simulink library "bcm"  (R2021b)
settings: Solver=VariableStepAuto  StartTime=0.0  StopTime=10.0  RelTol=1e-3
undefined symbols (not defined in the file or in its folder): ENUM_ANTITHEFT_ALARM, ENUM_ANTITHEFT_ARM, ENUM_ANTITHEFT_DISARM, ENUM_ANTITHEFT_WAIT, ENUM_GEARPOSNTOCAN_P, ENUM_PDKEYRAWLULOCK_INUNLOCK, ENUM_PDKEYRAWPS_INPS, ENUM_POWERSTA_ON, ENUM_POWERSTA_READY, ENUM_POWERSTA_STANDBY, FALSE, KBCM_ALMBrightnessDark_enum, KBCM_AmbBlue_enum, KBCM_AmbBreathT_ms, KBCM_AmbGreen_enum, KBCM_AmbRed_enum, KBCM_Antitheft_enum_ovrdflg, KBCM_Antitheft_enum_ovrdval, KBCM_APMDoorCtrlSta_flg_ovrdflg, KBCM_APMDoorCtrlSta_flg_ovrdval, KBCM_DelayTSW_flg, KBCM_DiagFLTC_mA, KBCM_DiagFMHT_s, KBCM_DiagFRTC_mA, KBCM_DiagRLTC_mA, KBCM_DiagRRTC_mA, KBCM_DrAPMRetryTimes_cnt, KBCM_DrOpenWdwOT_s, KBCM_DrOpenWdwReady_s, KBCM_ESSOffT_ms, KBCM_ESSOnT_ms, KBCM_IVIRstHoldT_ms, KBCM_IVIRstTriggerT_ms, KBCM_ONDelayT_ms, KBCM_ReDetectT_K, KBCM_RmLampKeep_min, KBCM_RmLpKeyInT_s, KBCM_RmLpKeyMissT_s, KBCM_SlpDebounceTime_s, KBCM_SPTGDetectT_sec, KBCM_SPTGLeave_flg, KBCM_SPTGLeftBound_cm, KBCM_SPTGLeftBoundOut_cm, KBCM_SPTGLowerBound_cm, KBCM_SPTGLowerBoundOut_cm, KBCM_SPTGRightBound_cm, KBCM_SPTGRightBoundOut_cm, KBCM_SPTGTOut_K, KBCM_SPTGUpperBound_cm, KBCM_SPTGUpperBoundOut_cm, KBCM_SPTGWaitDKC_sec, KBCM_TrunSWKeepTime3_s, KBCM_TrunSWKeepTime5_s, KBCM_TrunSWKeepTime7_s, KBCM_USSDis_cm, KBCM_USSFilterT_K, KBCM_WaitAPMPwr_K, KBCM_WdwManualDetT_s, MIN2SEC, TRUE ... (+1)
libraries: simulink x151, hcu_lib x5
(part 3 of 8)

== system bcm/BCM/BCM/APM_Door ==
  task_time_s : Inport
  VINP_OpenDrOpenWdoSW_flg : Inport  Port=2
  VINP_LDrvControlCommand_pct : Inport  Port=3
  VINP_LDrvValWdwOpened_pct : Inport  Port=4
  VINP_DrDoorSW_flg : Inport  Port=5
  VINP_LPasControlCommand_pct : Inport  Port=6
  VINP_LPasValWdwOpened_pct : Inport  Port=7
  VINP_PsDoorSW_flg : Inport  Port=8
  VINP_LRLDControlCommand_pct : Inport  Port=9
  VINP_LRLDValWdwOpened_pct : Inport  Port=10
  VINP_RLDoorSW_flg : Inport  Port=11
  VINP_LRRDControlCommand_pct : Inport  Port=12
  VINP_LRRDValWdwOpened_pct : Inport  Port=13
  VINP_RRDoorSW_flg : Inport  Port=14
  VINP_FlashAPMDoorControlSta_flg : Inport  Port=15
  BCMInitial : Inport  Port=16
  VINP_CANMsgValidIVI2_flg : Inport  Port=17
  VINP_CANMsgValidGWZoneDR1_flg : Inport  Port=18
  VINP_CANMsgValidGWZoneFR1_flg : Inport  Port=19
  Constant{,5..6,15} (4 alike) : Constant  Value=KBCM_WdwManualDetT_s
  Constant{1,3,7,10} (4 alike) : Constant  Value=KBCM_DrOpenWdwReady_s
  Constant{2,8,11,14} (4 alike) : Constant  Value=KBCM_WaitAPMPwr_K
  Constant{4,9,12..13} (4 alike) : Constant  Value=KBCM_DrOpenWdwOT_s
  Constant16 : Constant  Value=KBCM_APMDoorCtrlSta_flg_ovrdflg
  Constant17 : Constant  Value=KBCM_APMDoorCtrlSta_flg_ovrdval
  Constant{18..21} (4 alike) : Constant  Value=KBCM_DrAPMRetryTimes_cnt
  Data Type Conversion : DataTypeConversion  OutDataTypeStr=single
  Detect Increase : simulink/Logic and Bit Operations/Detect Increase  vinit=0.0  OutDataTypeStr=boolean
  DoorAPM : Subsystem
  DoorAPM1 : Subsystem
  DoorAPM2 : Subsystem
  DoorAPM3 : Subsystem
  NOT : Logic  Operator=NOT  AllPortsSameDT=off  OutDataTypeStr=boolean
  Switch : Switch  Criteria=u2 ~= 0
  Switch1 : Switch  Criteria=u2 ~= 0
  Switch9 : Switch  Criteria=u2 > Threshold
  Terminator{,1..3} (4 alike) : Terminator
  Unit Delay2 : UnitDelay  InitialCondition=1  SampleTime=-1  HasFrameUpgradeWarning=on
  VBCM_LDrvCtrlCmd_pct : Outport
  VBCM_LPasCtrlCmd_pct : Outport  Port=2
  VBCM_LRLDCtrlCmd_pct : Outport  Port=3
  VBCM_LRRDCtrlCmd_pct : Outport  Port=4
  VBCM_APMDoorControlSta_flg : Outport  Port=5
  wires:
  NOT/1 -> Switch/1
  VINP_OpenDrOpenWdoSW_flg/1 -> Detect Increase/1
  Detect Increase/1 -> Switch/2
  VINP_FlashAPMDoorControlSta_flg/1 -> Switch9/3
  Unit Delay2/1 -> NOT/1, Switch/3
  Switch/1 -> Switch9/1
  Switch9/1 -> Switch1/3, Unit Delay2/1
  task_time_s/1 -> Data Type Conversion/1
  [task_time_s] -> DoorAPM/1(task_time_s)
  [task_time_s] -> DoorAPM1/1(task_time_s)
  [task_time_s] -> DoorAPM2/1(task_time_s)
  [task_time_s] -> DoorAPM3/1(task_time_s)
  DoorAPM/1(CtrlCmd_pct) -> VBCM_LDrvCtrlCmd_pct/1  "VBCM_LDrvCtrlCmd_pct"
  DoorAPM1/1(CtrlCmd_pct) -> VBCM_LPasCtrlCmd_pct/1  "VBCM_LPasCtrlCmd_pct"
  DoorAPM2/1(CtrlCmd_pct) -> VBCM_LRLDCtrlCmd_pct/1  "VBCM_LRLDCtrlCmd_pct"
  DoorAPM3/1(CtrlCmd_pct) -> VBCM_LRRDCtrlCmd_pct/1  "VBCM_LRRDCtrlCmd_pct"
  DoorAPM/2(CtrlCmdReady_flg) -> Terminator/1  "VBCM_LDrvCtrlCmdReady_flg"
  DoorAPM1/2(CtrlCmdReady_flg) -> Terminator1/1  "VBCM_LPasCtrlCmdReady_flg"
  DoorAPM2/2(CtrlCmdReady_flg) -> Terminator2/1  "VBCM_LRLDCtrlCmdReady_flg"
  DoorAPM3/2(CtrlCmdReady_flg) -> Terminator3/1  "VBCM_LRRDCtrlCmdReady_flg"
  Switch1/1 -> [VBCM_APMDoorControlSta_flg], VBCM_APMDoorControlSta_flg/1  "VBCM_APMDoorControlSta_flg"
  Constant16/1 -> Switch1/2
  Constant17/1 -> Switch1/1
  VINP_CANMsgValidIVI2_flg/1 -> [VINP_CANMsgValidIVI2_flg]
  VINP_CANMsgValidGWZoneDR1_flg/1 -> [VINP_CANMsgValidGWZoneDR1_flg]
  VINP_CANMsgValidGWZoneFR1_flg/1 -> [VINP_CANMsgValidGWZoneFR1_flg]
  [VINP_CANMsgValidGWZoneFR1_flg] -> DoorAPM/12(CANMsgValidGWZoneFR1)
  [VINP_CANMsgValidGWZoneDR1_flg] -> DoorAPM/11(CANMsgValidGWZoneDR1)
  [VBCM_APMDoorControlSta_flg] -> DoorAPM/5(APMDoorControlSta_flg)
  Constant8/1 -> DoorAPM/6(WaitAPMPwr_K)
  Constant9/1 -> DoorAPM/7(DrOpenWdwOT_s)
  Constant7/1 -> DoorAPM/8(DrOpenWdwReady_s)
  Constant18/1 -> DoorAPM/13(KBCM_DrAPMRetryTimes_cnt)
  Constant/1 -> DoorAPM/9(KBCM_WdwManualDetT_K)
  [VINP_CANMsgValidIVI2_flg] -> DoorAPM/10(CANMsgValidIVI2)
  VINP_DrDoorSW_flg/1 -> DoorAPM/2(DoorSW_flg)
  VINP_LDrvControlCommand_pct/1 -> DoorAPM/3(ControlCommand_pct)
  VINP_LDrvValWdwOpened_pct/1 -> DoorAPM/4(ValWdwOpened_pct)
  [VINP_CANMsgValidGWZoneDR1_flg] -> DoorAPM1/11(CANMsgValidGWZoneDR1)
  [VINP_CANMsgValidGWZoneFR1_flg] -> DoorAPM1/12(CANMsgValidGWZoneFR1)
  [VBCM_APMDoorControlSta_flg] -> DoorAPM1/5(APMDoorControlSta_flg)
  Constant11/1 -> DoorAPM1/6(WaitAPMPwr_K)
  Constant12/1 -> DoorAPM1/7(DrOpenWdwOT_s)
  Constant10/1 -> DoorAPM1/8(DrOpenWdwReady_s)
  Constant5/1 -> DoorAPM1/9(KBCM_WdwManualDetT_K)
  [VINP_CANMsgValidIVI2_flg] -> DoorAPM1/10(CANMsgValidIVI2)
  Constant19/1 -> DoorAPM1/13(KBCM_DrAPMRetryTimes_cnt)
  VINP_PsDoorSW_flg/1 -> DoorAPM1/2(DoorSW_flg)
  VINP_LPasControlCommand_pct/1 -> DoorAPM1/3(ControlCommand_pct)
  VINP_LPasValWdwOpened_pct/1 -> DoorAPM1/4(ValWdwOpened_pct)
  [VINP_CANMsgValidGWZoneDR1_flg] -> DoorAPM2/11(CANMsgValidGWZoneDR1)
  [VINP_CANMsgValidGWZoneFR1_flg] -> DoorAPM2/12(CANMsgValidGWZoneFR1)
  [VBCM_APMDoorControlSta_flg] -> DoorAPM2/5(APMDoorControlSta_flg)
  Constant2/1 -> DoorAPM2/6(WaitAPMPwr_K)
  Constant13/1 -> DoorAPM2/7(DrOpenWdwOT_s)
  Constant1/1 -> DoorAPM2/8(DrOpenWdwReady_s)
  Constant6/1 -> DoorAPM2/9(KBCM_WdwManualDetT_K)
  [VINP_CANMsgValidIVI2_flg] -> DoorAPM2/10(CANMsgValidIVI2)
  Constant20/1 -> DoorAPM2/13(KBCM_DrAPMRetryTimes_cnt)
  VINP_RLDoorSW_flg/1 -> DoorAPM2/2(DoorSW_flg)
  VINP_LRLDControlCommand_pct/1 -> DoorAPM2/3(ControlCommand_pct)
  VINP_LRLDValWdwOpened_pct/1 -> DoorAPM2/4(ValWdwOpened_pct)
  [VINP_CANMsgValidGWZoneDR1_flg] -> DoorAPM3/11(CANMsgValidGWZoneDR1)
  [VINP_CANMsgValidGWZoneFR1_flg] -> DoorAPM3/12(CANMsgValidGWZoneFR1)
  [VBCM_APMDoorControlSta_flg] -> DoorAPM3/5(APMDoorControlSta_flg)
  Constant14/1 -> DoorAPM3/6(WaitAPMPwr_K)
  Constant4/1 -> DoorAPM3/7(DrOpenWdwOT_s)
  Constant3/1 -> DoorAPM3/8(DrOpenWdwReady_s)
  Constant15/1 -> DoorAPM3/9(KBCM_WdwManualDetT_K)
  [VINP_CANMsgValidIVI2_flg] -> DoorAPM3/10(CANMsgValidIVI2)
  Constant21/1 -> DoorAPM3/13(KBCM_DrAPMRetryTimes_cnt)
  VINP_RRDoorSW_flg/1 -> DoorAPM3/2(DoorSW_flg)
  VINP_LRRDControlCommand_pct/1 -> DoorAPM3/3(ControlCommand_pct)
  VINP_LRRDValWdwOpened_pct/1 -> DoorAPM3/4(ValWdwOpened_pct)
  Data Type Conversion/1 -> [task_time_s]
  BCMInitial/1 -> Switch9/2

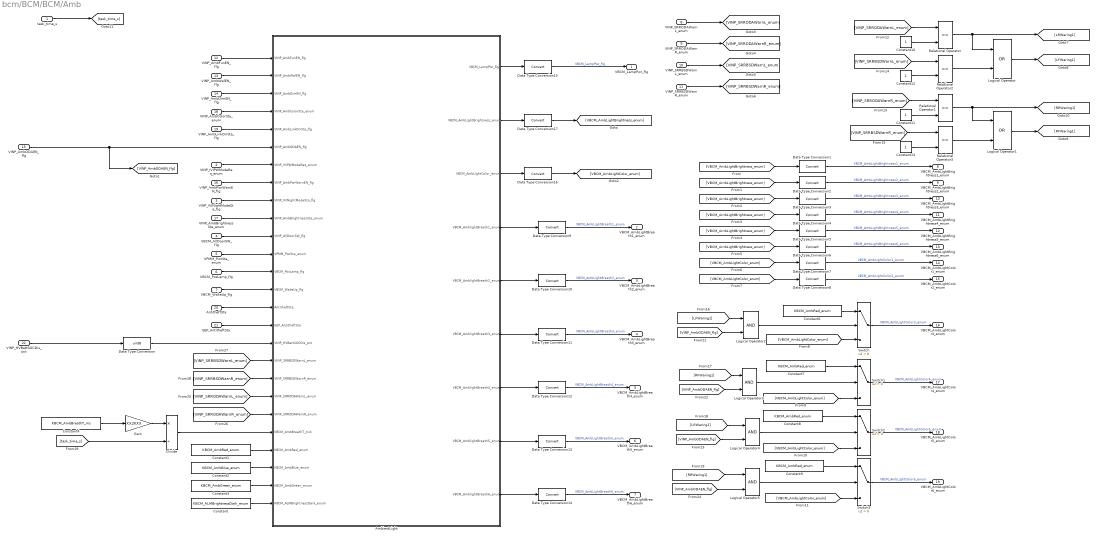
== system bcm/BCM/BCM/Amb ==
  task_time_s : Inport
  VINP_IVIPWModeReq_enum : Inport  Port=2
  VINP_IVINightModeSta_flg : Inport  Port=3
  VBCM_AllDoorSW_flg : Inport  Port=4
  VPMM_PwrSta_enum : Inport  Port=5
  VBCM_PosLamp_flg : Inport  Port=6
  VBCM_WakeUp_flg : Inport  Port=7
  VINP_SRRODAWarnL_enum : Inport  Port=8
  VINP_SRRODAWarnR_enum : Inport  Port=9
  VINP_SRRBSDWarnL_enum : Inport  Port=10
  VINP_SRRBSDWarnR_enum : Inport  Port=11
  VINP_AmbFunEN_flg : Inport  Port=12
  VINP_AmbWelEN_flg : Inport  Port=13
  VINP_AmbDimEN_flg : Inport  Port=14
  VINP_AmbODAEN_flg : Inport  Port=15
  VINP_AmbPwrWarnEN_flg : Inport  Port=16
  VINP_AmbBrightnessSta_enum : Inport  Port=17
  VINP_AmbColorSta_enum : Inport  Port=18
  VINP_AmbLinkDriSta_flg : Inport  Port=19
  AntitheftSta : Inport  Port=20
  EEP_AntitheftSta : Inport  Port=21
  VINP_HVBattSOCDis_pct : Inport  Port=22
  AmbientLight : Stateflow chart  TreatAsAtomicUnit=on
      settings: PortSchema="{\"entries\":[{\"content\":{\"sides\":[{\"content\":{\"connectorIds\":[\"In4\",\"In1\",\"In3\",\"In2\",\"In11\",\"In6\",\"In12\",\"In8\",\"In15\",\"In10\",\"In17\",\"In18\",\"In16\",\"In19\",\"In20\",\"In21\",\"In22\",\"In23\",\"In24\",\"In25\",\"In26\",\"In14\",\"In9\",\"In13\",\"In7\",\"In5\"]},\"type\":\"ConnectorPlacement.EquallySpacedRectSide\",\"uuid\":\"e6ddbb92-6bab-4ee4-8600-41e59bb8ed99\"},{\"content\":{\"connectorIds\":[\"Out1\",\"Out2\",\"Out3\",\"Out4\",\"Out5\",\"Out6\",\"Out7\",\"Out8\",\"Out9\"],\"side\":\"RIGHT\"},\"type\":\"ConnectorPlacement.EquallySpacedRectSide\",\"uuid\":\"8a02ea17-d632-4a57-b5aa-65195147745e\"},{\"content\":{\"side\":\"TOP\"},\"type\":\"ConnectorPlacement.EquallySpacedRectSide\",\"uuid\":\"3394b4a4-a92c-4aad-9aa4-5f4e7dfad0c8\"}]},\"type\":\"ConnectorPlacement.EquallySpacedConnector\",\"uuid\":\"350d749b-651a-4475-8984-e64d423840e0\"}],\"packageUris\":[\"http://schema.mathworks.com/mf0/Connector/R2020b\"],\"version\":\"1.0\"}"
  Constant : Constant  Value=KBCM_ALMBrightnessDark_enum  OutDataTypeStr=uint8
  Constant{1,6..9} (5 alike) : Constant  Value=KBCM_AmbRed_enum  OutDataTypeStr=uint8
  Constant{10..13} (4 alike) : Constant
  Constant2 : Constant  Value=KBCM_AmbBlue_enum  OutDataTypeStr=uint8
  Constant3 : Constant  Value=KBCM_AmbGreen_enum  OutDataTypeStr=uint8
  Constant4 : Constant  Value=KBCM_AmbBreathT_ms
  Data Type Conversion : DataTypeConversion  OutDataTypeStr=uint8
  Data Type Conversion{1..17} (17 alike) : DataTypeConversion
  Divide : Product  Inputs=*/
  Gain : Gain  Gain=XX2KXX
  Logical Operator : Logic  Operator=OR  AllPortsSameDT=off  OutDataTypeStr=boolean
  Logical Operator1 : Logic  Operator=OR  AllPortsSameDT=off  OutDataTypeStr=boolean
  Logical Operator{2..5} (4 alike) : Logic  AllPortsSameDT=off  OutDataTypeStr=boolean
  Relational Operator{,1..3} (4 alike) : RelationalOperator  Operator===  OutDataTypeStr=boolean  RndMeth=Simplest
  Switch{,1..3} (4 alike) : Switch  Criteria=u2 > Threshold
  VBCM_LampPwr_flg : Outport
  VBCM_AmbLightBreath1_enum : Outport  Port=2
  VBCM_AmbLightBreath2_enum : Outport  Port=3
  VBCM_AmbLightBreath3_enum : Outport  Port=4
  VBCM_AmbLightBreath4_enum : Outport  Port=5
  VBCM_AmbLightBreath5_enum : Outport  Port=6
  VBCM_AmbLightBreath6_enum : Outport  Port=7
  VBCM_AmbLightBrightness1_enum : Outport  Port=8
  VBCM_AmbLightBrightness2_enum : Outport  Port=9
  VBCM_AmbLightBrightness3_enum : Outport  Port=10
  VBCM_AmbLightBrightness4_enum : Outport  Port=11
  VBCM_AmbLightBrightness5_enum : Outport  Port=12
  VBCM_AmbLightBrightness6_enum : Outport  Port=13
  VBCM_AmbLightColor1_enum : Outport  Port=14
  VBCM_AmbLightColor2_enum : Outport  Port=15
  VBCM_AmbLightColor3_enum : Outport  Port=16
  VBCM_AmbLightColor4_enum : Outport  Port=17
  VBCM_AmbLightColor5_enum : Outport  Port=18
  VBCM_AmbLightColor6_enum : Outport  Port=19
  wires:
  [RRWaring1] -> Logical Operator5/1
  VINP_SRRBSDWarnR_enum/1 -> [VINP_SRRBSDWarnR_enum]
  Relational Operator3/1 -> Logical Operator1/2
  [VBCM_AmbLightColor_enum] -> Switch/3
  Relational Operator/1 -> [LRWaring1], Logical Operator/1
  [VINP_AmbODAEN_flg] -> Logical Operator3/2
  [VINP_SRRBSDWarnR_enum] -> Relational Operator3/1
  Constant8/1 -> Switch2/1
  [VBCM_AmbLightBrightness_enum] -> Data Type Conversion2/1
  Constant11/1 -> Relational Operator1/2
  Constant10/1 -> Relational Operator/2
  [VBCM_AmbLightBrightness_enum] -> Data Type Conversion4/1
  [VINP_AmbODAEN_flg] -> Logical Operator4/2
  Logical Operator4/1 -> Switch2/2
  [VINP_SRRBSDWarnL_enum] -> Relational Operator2/1
  AmbientLight/3(VBCM_AmbLightColor_enum) -> Data Type Conversion16/1
  [VINP_SRRODAWarnL_enum] -> AmbientLight/25(VINP_SRRODAWarnL_enum)
  [RFWaring1] -> Logical Operator3/1
  [VINP_SRRODAWarnR_enum] -> AmbientLight/26(VINP_SRRODAWarnR_enum)
  [VINP_AmbODAEN_flg] -> Logical Operator2/2
  Switch3/1 -> VBCM_AmbLightColor6_enum/1  "VBCM_AmbLightColor6_enum"
  VINP_SRRODAWarnR_enum/1 -> [VINP_SRRODAWarnR_enum]
  [LFWaring1] -> Logical Operator2/1
  [VBCM_AmbLightColor_enum] -> Switch1/3
  [VINP_SRRBSDWarnL_enum] -> AmbientLight/23(VINP_SRRBSDWarnL_enum)
  [VBCM_AmbLightBrightness_enum] -> Data Type Conversion6/1
  VBCM_PosLamp_flg/1 -> AmbientLight/16(VBCM_PosLamp_flg)
  VINP_SRRODAWarnL_enum/1 -> [VINP_SRRODAWarnL_enum]
  Constant1/1 -> AmbientLight/9(KBCM_AmbRed_enum)
  Logical Operator5/1 -> Switch3/2
  [VBCM_AmbLightColor_enum] -> Switch3/3
  Switch1/1 -> VBCM_AmbLightColor4_enum/1  "VBCM_AmbLightColor4_enum"
  Logical Operator3/1 -> Switch1/2
  Relational Operator1/1 -> Logical Operator1/1, [RRWaring1]
  VBCM_WakeUp_flg/1 -> AmbientLight/19(VBCM_WakeUp_flg)
  [VINP_SRRBSDWarnR_enum] -> AmbientLight/24(VINP_SRRBSDWarnR_enum)
  [VINP_SRRODAWarnR_enum] -> Relational Operator1/1
  Constant9/1 -> Switch3/1
  AmbientLight/8(VBCM_AmblightBreath5_enum) -> Data Type Conversion13/1
  AmbientLight/1(VBCM_LampPwr_flg) -> Data Type Conversion15/1
  Constant2/1 -> AmbientLight/13(KBCM_AmbBlue_enum)
  Constant13/1 -> Relational Operator3/2
  Constant3/1 -> AmbientLight/7(KBCM_AmbGreen_enum)
  Constant6/1 -> Switch/1
  AmbientLight/9(VBCM_AmblightBreath6_enum) -> Data Type Conversion14/1
  [VBCM_AmbLightColor_enum] -> Switch2/3
  [VBCM_AmbLightBrightness_enum] -> Data Type Conversion3/1
  VINP_SRRBSDWarnL_enum/1 -> [VINP_SRRBSDWarnL_enum]
  [VBCM_AmbLightBrightness_enum] -> Data Type Conversion5/1
  AmbientLight/7(VBCM_AmblightBreath4_enum) -> Data Type Conversion12/1
  Relational Operator2/1 -> Logical Operator/2
  AmbientLight/6(VBCM_AmblightBreath3_enum) -> Data Type Conversion11/1
  Logical Operator1/1 -> [RFWaring1]
  Logical Operator/1 -> [LFWaring1]
  Constant7/1 -> Switch1/1
  [VBCM_AmbLightColor_enum] -> Data Type Conversion7/1
  [VBCM_AmbLightColor_enum] -> Data Type Conversion8/1
  [VINP_SRRODAWarnL_enum] -> Relational Operator/1
  EEP_AntitheftSta/1 -> AmbientLight/21(EEP_AntitheftSta)
  Logical Operator2/1 -> Switch/2
  VINP_HVBattSOCDis_pct/1 -> Data Type Conversion/1
  Constant12/1 -> Relational Operator2/2
  Switch/1 -> VBCM_AmbLightColor3_enum/1  "VBCM_AmbLightColor3_enum"
  [VINP_AmbODAEN_flg] -> Logical Operator5/2
  Switch2/1 -> VBCM_AmbLightColor5_enum/1  "VBCM_AmbLightColor5_enum"
  AntitheftSta/1 -> AmbientLight/20(AntitheftSta)
  [LRWaring1] -> Logical Operator4/1
  VPMM_PwrSta_enum/1 -> AmbientLight/18(VPMM_PwrSta_enum)
  VBCM_AllDoorSW_flg/1 -> AmbientLight/17(VINP_AllDoorSW_flg)
  AmbientLight/5(VBCM_AmblightBreath2_enum) -> Data Type Conversion10/1
  [VBCM_AmbLightBrightness_enum] -> Data Type Conversion1/1
  AmbientLight/4(VBCM_AmblightBreath1_enum) -> Data Type Conversion9/1
  Constant/1 -> AmbientLight/5(KBCM_ALMBrightnessDark_enum)
  [task_time_s] -> Divide/2
  Gain/1 -> Divide/1
  Constant4/1 -> Gain/1
  Divide/1 -> AmbientLight/14(KBCM_AmbBreathT_tick)
  task_time_s/1 -> [task_time_s]
  VINP_AmbFunEN_flg/1 -> AmbientLight/4(VINP_AmbFunEN_flg)
  VINP_AmbWelEN_flg/1 -> AmbientLight/1(VINP_AmbWelEN_flg)
  VINP_AmbDimEN_flg/1 -> AmbientLight/3(VINP_AmbDimEN_flg)
  VINP_AmbColorSta_enum/1 -> AmbientLight/2(VINP_AmbColorSta_enum)
  VINP_AmbLinkDriSta_flg/1 -> AmbientLight/11(VINP_AmbLinkDriSta_flg)
  VINP_AmbODAEN_flg/1 -> [VINP_AmbODAEN_flg], AmbientLight/6(VINP_AmbODAEN_flg)
  VINP_IVIPWModeReq_enum/1 -> AmbientLight/12(VINP_IVIPWModeReq_enum)
  VINP_AmbPwrWarnEN_flg/1 -> AmbientLight/8(VINP_AmbPwrWarnEN_flg)
  VINP_IVINightModeSta_flg/1 -> AmbientLight/15(VINP_IVINightModeSta_flg)
  VINP_AmbBrightnessSta_enum/1 -> AmbientLight/10(VINP_AmbBrightnessSta_enum)
  Data Type Conversion/1 -> AmbientLight/22(VINP_HVBattSOCDis_pct)
  Data Type Conversion1/1 -> VBCM_AmbLightBrightness1_enum/1  "VBCM_AmbLightBrightness1_enum"
  Data Type Conversion2/1 -> VBCM_AmbLightBrightness2_enum/1  "VBCM_AmbLightBrightness2_enum"
  Data Type Conversion3/1 -> VBCM_AmbLightBrightness3_enum/1  "VBCM_AmbLightBrightness3_enum"
  Data Type Conversion4/1 -> VBCM_AmbLightBrightness4_enum/1  "VBCM_AmbLightBrightness4_enum"
  Data Type Conversion5/1 -> VBCM_AmbLightBrightness5_enum/1  "VBCM_AmbLightBrightness5_enum"
  Data Type Conversion6/1 -> VBCM_AmbLightBrightness6_enum/1  "VBCM_AmbLightBrightness6_enum"
  Data Type Conversion7/1 -> VBCM_AmbLightColor1_enum/1  "VBCM_AmbLightColor1_enum"
  Data Type Conversion8/1 -> VBCM_AmbLightColor2_enum/1  "VBCM_AmbLightColor2_enum"
  Data Type Conversion9/1 -> VBCM_AmbLightBreath1_enum/1  "VBCM_AmbLightBreath1_enum"
  Data Type Conversion10/1 -> VBCM_AmbLightBreath2_enum/1  "VBCM_AmbLightBreath2_enum"
  Data Type Conversion11/1 -> VBCM_AmbLightBreath3_enum/1  "VBCM_AmbLightBreath3_enum"
  Data Type Conversion12/1 -> VBCM_AmbLightBreath4_enum/1  "VBCM_AmbLightBreath4_enum"
  Data Type Conversion13/1 -> VBCM_AmbLightBreath5_enum/1  "VBCM_AmbLightBreath5_enum"
  Data Type Conversion14/1 -> VBCM_AmbLightBreath6_enum/1  "VBCM_AmbLightBreath6_enum"
  Data Type Conversion15/1 -> VBCM_LampPwr_flg/1  "VBCM_LampPwr_flg"
  Data Type Conversion16/1 -> [VBCM_AmbLightColor_enum]
  AmbientLight/2(VBCM_AmbLightBrightness_enum) -> Data Type Conversion17/1
  Data Type Conversion17/1 -> [VBCM_AmbLightBrightness_enum]

== system bcm/BCM/BCM/AntiTheft ==
  VINP_PCommandToBCM_enum : Inport
  VPMM_PwrSta_enum : Inport  Port=2
  VINP_HoodSW_flg : Inport  Port=3
  VINP_TailgateSW_flg : Inport  Port=4
  VINP_DrDoorSW_flg : Inport  Port=5
  VINP_PsDoorSW_flg : Inport  Port=6
  VINP_RLDoorSW_flg : Inport  Port=7
  VINP_RRDoorSW_flg : Inport  Port=8
  VINP_DrLockSta_flg : Inport  Port=9
  VINP_ReDoorLock_enum : Inport  Port=10
  VINP_VehSpeed_kph : Inport  Port=11
  VBCM_fVIGHandle_flg : Inport  Port=12
  VBCM_FlashAntitheft_enum : Inport  Port=13
  VINP_APSOpenPTG_flg : Inport  Port=14
  VINP_FlashCountAlarm_enum : Inport  Port=15
  VINP_CANMsgValidGWZoneDR1_flg : Inport  Port=16
  VINP_CANMsgValidGWZoneFR1_flg : Inport  Port=17
  VINP_CANMsgValidIVI1_flg : Inport  Port=18
  VINP_IVILockSoundSWSta_flg : Inport  Port=19
  Antitheft__override : Subsystem
  Chart : Stateflow chart  TreatAsAtomicUnit=on
  Data Type Conversion : DataTypeConversion  OutDataTypeStr=uint8
  Data Type Conversion1 : DataTypeConversion  OutDataTypeStr=boolean
  Logical Operator : Logic  Operator=OR  Inputs=4  AllPortsSameDT=off  OutDataTypeStr=boolean
  Switch : Switch  Criteria=u2 ~= 0
  Unit Delay : UnitDelay  SampleTime=-1  HasFrameUpgradeWarning=on
  VIG_Decoder : MATLAB Function  TreatAsAtomicUnit=on
  VBCM_ATCtrl_enum : Outport
  VBCM_ATActCtrl_enum : Outport  Port=2
  VBCM_ATAlarm_flg : Outport  Port=3
  VBCM_AntitheftSta_enum : Outport  Port=4
  VBCM_TailgateRemote_enum : Outport  Port=5
  VBCM_HornCtrl_flg : Outport  Port=6
  VBCM_AllDoorSW_flg : Outport  Port=7
  VBCM_BCMDoorLockSta_flg : Outport  Port=8
  VBCM_AntitehftSeatFlod_flg : Outport  Port=9
  VBCM_HoodSW_flg : Outport  Port=10
  VBCM_TailgateSW_flg : Outport  Port=11
  VBCM_DrDoorSW_flg : Outport  Port=12
  VBCM_PsDoorSW_flg : Outport  Port=13
  VBCM_RLDoorSW_flg : Outport  Port=14
  VBCM_RRDoorSW_flg : Outport  Port=15
  VBCM_CountAlarm_enum : Outport  Port=16
  VBCM_LockAlarm_enum : Outport  Port=17
  wires:
  VBCM_fVIGHandle_flg/1 -> Chart/13(fVIGHandle)  "VBCM_fVIGHandle_flg"
  VINP_RRDoorSW_flg/1 -> [RRDoorSW]
  VINP_ReDoorLock_enum/1 -> VIG_Decoder/1(VINP_ReDoorLock_enum)
  Chart/2(ATLockCtrl) -> VBCM_ATActCtrl_enum/1  "VBCM_ATActCtrl_enum"
  Chart/1(ATCtrl) -> VBCM_ATCtrl_enum/1  "VBCM_ATCtrl_enum"
  VINP_PCommandToBCM_enum/1 -> Chart/1(P_CommandtoBCM)
  VINP_RLDoorSW_flg/1 -> [RLDoorSW]
  Chart/3(ATAlarm) -> VBCM_ATAlarm_flg/1  "VBCM_ATAlarm_flg"
  VINP_PsDoorSW_flg/1 -> [PsDoorSW]
  VINP_VehSpeed_kph/1 -> Chart/12(VehSpeed)  "VINP_VehSpeed_kph"
  Logical Operator/1 -> [VBCM_AllDoorSW_flg]  "VBCM_AllDoorSW_flg"
  VINP_DrDoorSW_flg/1 -> [DrDoorSW]
  VINP_HoodSW_flg/1 -> [HoodSW]
  VIG_Decoder/1(VIG_Cmd) -> Data Type Conversion/1
  Data Type Conversion/1 -> Chart/11(VIG_Cmd)  "VBCM_VIGCommand_enum"
  [VBCM_AllDoorSW_flg] -> VBCM_AllDoorSW_flg/1  "VBCM_AllDoorSW_flg"
  Chart/4(AntitheftSta) -> Antitheft__override/1(In1)  "VBCM_AntitheftSta_enum"
  Chart/5(TailgateRemote) -> VBCM_TailgateRemote_enum/1  "VBCM_TailgateRemote_enum"
  Chart/6(HornCtrl) -> VBCM_HornCtrl_flg/1  "VBCM_HornCtrl_flg"
  Chart/7(AntitheftSeatFlod) -> VBCM_AntitehftSeatFlod_flg/1  "VBCM_AntitheftSeatFlod_flg"
  Antitheft__override/1(Out1) -> VBCM_AntitheftSta_enum/1  "VBCM_AntitheftSta_enum"
  VINP_APSOpenPTG_flg/1 -> Chart/15(APSOpenPTG)  "VINP_APSOpenPTG_flg"
  VINP_TailgateSW_flg/1 -> [TailgateSW]
  [DrDoorSW] -> Logical Operator/1
  [PsDoorSW] -> Logical Operator/2
  [RLDoorSW] -> Logical Operator/3
  [RRDoorSW] -> Logical Operator/4
  VINP_DrLockSta_flg/1 -> [DrLockSta]
  [DrLockSta] -> VBCM_BCMDoorLockSta_flg/1  "VBCM_BCMDoorLockSta_flg"
  [HoodSW] -> VBCM_HoodSW_flg/1  "VBCM_HoodSW_flg"
  [TailgateSW] -> VBCM_TailgateSW_flg/1  "VBCM_TailgateSW_flg"
  [DrDoorSW] -> VBCM_DrDoorSW_flg/1  "VBCM_DrDoorSW_flg"
  [PsDoorSW] -> VBCM_PsDoorSW_flg/1  "VBCM_PsDoorSW_flg"
  [RLDoorSW] -> VBCM_RLDoorSW_flg/1  "VBCM_RLDoorSW_flg"
  [RRDoorSW] -> VBCM_RRDoorSW_flg/1  "VBCM_RRDoorSW_flg"
  VPMM_PwrSta_enum/1 -> Chart/2(PwrSta)
  VBCM_FlashAntitheft_enum/1 -> Chart/14(VBCM_FlashAntitheft_enum)
  [DrDoorSW] -> Chart/6(DrDoorSW)
  [TailgateSW] -> Chart/5(TailgateSW)
  [PsDoorSW] -> Chart/7(PsDoorSW)
  [HoodSW] -> Chart/4(HoodSW)
  [RRDoorSW] -> Chart/9(RRDoorSW)
  [RLDoorSW] -> Chart/8(RLDoorSW)
  [DrLockSta] -> Chart/10(DrLockSta)
  [VBCM_AllDoorSW_flg] -> Chart/3(AllDoorSW)
  VINP_FlashCountAlarm_enum/1 -> Chart/16(VINP_FlashCountAlarm_enum)
  VINP_CANMsgValidGWZoneDR1_flg/1 -> Chart/17(VINP_CANMsgValidGWZoneDR1_flg)
  VINP_CANMsgValidGWZoneFR1_flg/1 -> Chart/18(VINP_CANMsgValidGWZoneFR1_flg)
  Chart/8(CountAlarm) -> VBCM_CountAlarm_enum/1  "VBCM_CountAlarm_enum"
  VINP_IVILockSoundSWSta_flg/1 -> Switch/1
  Switch/1 -> Data Type Conversion1/1, Unit Delay/1
  VINP_CANMsgValidIVI1_flg/1 -> Switch/2
  Unit Delay/1 -> Switch/3
  Chart/9(VBCM_LockAlarm_enum) -> VBCM_LockAlarm_enum/1  "VBCM_LockAlarm_enum"
  Data Type Conversion1/1 -> Chart/19(IVI_Lock_SoundSW_Sta)

== system bcm/BCM/BCM/BCM_WAKE_MODULE ==
  note: SIMULINK_BASED
  note: STATEFLOW_BASED
  note: The initial value of this uint dealy is "1"
  VBCM_HoodSW_flg : Inport
  VBCM_TailgateSW_flg : Inport  Port=2
  VBCM_CTDLockSW_flg : Inport  Port=3
  VBCM_TailgateHDSW_flg : Inport  Port=4
  VBCM_AntitheftSta_enum : Inport  Port=5
  VBCM_AllDoorSW_flg : Inport  Port=6
  VBCM_HornCtrl_flg : Inport  Port=7
  VBCM_DoorLockIND_flg : Inport  Port=8
  VINP_BrakeSWGPIO_flg : Inport  Port=9
  VBCM_PosLamp_flg : Inport  Port=10
  VBCM_LBSD_flg : Inport  Port=11
  VBCM_RBSD_flg : Inport  Port=12
  VBCM_LTurnLP_flg : Inport  Port=13
  VBCM_RTurnLP_flg : Inport  Port=14
  VBCM_MirrorCtrl_enum : Inport  Port=15
  VBCM_RoomLampH_flg : Inport  Port=16
  task_time_s : Inport  Port=17
  VINP_FlashHoodSW_flg : Inport  Port=18
  VINP_FlashTailgateSW_flg : Inport  Port=19
  VINP_FlashCTDLockSW_flg : Inport  Port=20
  VINP_FlashTailgateHDSW_flg : Inport  Port=21
  Chart : Stateflow chart  TreatAsAtomicUnit=on
  Compare To Constant : simulink/Logic and Bit Operations/Compare To Constant  relop=>  const=0  OutDataTypeStr=boolean
  Constant : Constant  Value=TRUE
  Constant1 : Constant  Commented=on  Value=TRUE
  Constant2 : Constant  Value=KBCM_SlpDebounceTime_s
  Constant5 : Constant  Commented=on  Value=KBCM_SlpDebounceTime_s
  Data Type Conversion : DataTypeConversion
  Detect Change : simulink/Logic and Bit Operations/Detect Change  vinit=0  OutDataTypeStr=boolean
  Detect Increase{,1..4} (5 alike) : simulink/Logic and Bit Operations/Detect Increase  vinit=0.0  OutDataTypeStr=boolean
  From : From  Commented=on  GotoTag=VBCM_SleepReq_flg
  From1 : From  Commented=on  GotoTag=VBCM_SlpConditionMeet_flg
  From2 : From  Commented=on  GotoTag=VBCM_SlpConditionMeet_flg
  From4 : From  Commented=on  GotoTag=task_time_s
  Goto : Goto  Commented=on  GotoTag=VBCM_SleepReq_flg
  Goto11 : Goto  Commented=on  GotoTag=VBCM_WakeUp_flg
  GreaterThan{,1..3} (4 alike) : RelationalOperator  Operator=>  OutDataTypeStr=boolean  RndMeth=Simplest
  GreaterThanOrEqual : RelationalOperator  Commented=on  OutDataTypeStr=boolean  RndMeth=Simplest
  Logical Operator : Logic  Operator=OR  Inputs=16  AllPortsSameDT=off  OutDataTypeStr=boolean
  Logical Operator{1,6..9} (5 alike) : Logic  AllPortsSameDT=off  OutDataTypeStr=boolean
  Logical Operator10 : Logic  Operator=NOT  AllPortsSameDT=off  OutDataTypeStr=boolean
  Logical Operator2 : Logic  Commented=on  AllPortsSameDT=off  OutDataTypeStr=boolean
  Logical Operator3 : Logic  Commented=on  Operator=NOT  AllPortsSameDT=off  OutDataTypeStr=boolean
  Logical Operator4 : Logic  Operator=NOT  AllPortsSameDT=off  OutDataTypeStr=boolean
  Logical Operator5 : Logic  Commented=on  Operator=NOT  AllPortsSameDT=off  OutDataTypeStr=boolean
  Switch : Switch  Commented=on  Criteria=u2 > Threshold
  Timer : hcu_lib/Basic_Blocks/Timer  Commented=on
  Udelay_Init_ONE : UnitDelay  Commented=on  InitialCondition=1  SampleTime=-1  HasFrameUpgradeWarning=on
  Unit Delay : UnitDelay  SampleTime=-1  HasFrameUpgradeWarning=on
  VBCM_SleepReq_flg : Outport
  VBCM_WakeUp_flg : Outport  Port=2
  wires:
  VBCM_DoorLockIND_flg/1 -> Logical Operator/8
  VBCM_LBSD_flg/1 -> Logical Operator/11
  VBCM_RoomLampH_flg/1 -> Logical Operator/16
  VBCM_RBSD_flg/1 -> Logical Operator/12
  VBCM_HornCtrl_flg/1 -> Logical Operator/7
  VBCM_AllDoorSW_flg/1 -> Detect Increase/1
  VBCM_RTurnLP_flg/1 -> Logical Operator/14
  Compare To Constant/1 -> Logical Operator/15
  VBCM_PosLamp_flg/1 -> Logical Operator/10
  VINP_BrakeSWGPIO_flg/1 -> Logical Operator/9
  VBCM_MirrorCtrl_enum/1 -> Compare To Constant/1
  VBCM_LTurnLP_flg/1 -> Logical Operator/13
  Detect Change/1 -> Logical Operator1/1
  VBCM_AntitheftSta_enum/1 -> Detect Change/1
  Constant5/1 -> GreaterThanOrEqual/2, Timer/4
  Timer/1 -> GreaterThanOrEqual/1
  Logical Operator/1 -> Logical Operator4/1
  Logical Operator1/1 -> Logical Operator/5
  Unit Delay/1 -> Logical Operator1/2
  Constant/1 -> Unit Delay/1
  Logical Operator4/1 -> [VBCM_SlpConditionMeet_flg]
  Switch/1 -> Logical Operator3/1, Goto/1  "VBCM_SleepReq_flg"
  Logical Operator2/1 -> Switch/2
  Constant1/1 -> Switch/1
  From/1 -> Udelay_Init_ONE/1
  GreaterThanOrEqual/1 -> Switch/3
  Udelay_Init_ONE/1 -> Logical Operator2/1
  Logical Operator5/1 -> Timer/2
  From2/1 -> Logical Operator2/2
  From1/1 -> Logical Operator5/1, Timer/1
  task_time_s/1 -> [task_time_s]
  From4/1 -> Timer/3
  VBCM_HoodSW_flg/1 -> [VBCM_HoodSW_flg]
  [VINP_FlashHoodSW_flg] -> GreaterThan/2
  GreaterThan/1 -> Logical Operator6/2
  Logical Operator6/1 -> Logical Operator/1
  [VBCM_HoodSW_flg] -> GreaterThan/1, Detect Increase4/1
  Detect Increase4/1 -> Logical Operator6/1
  VBCM_TailgateSW_flg/1 -> [VBCM_TailgateSW_flg]
  [VBCM_CTDLockSW_flg] -> Detect Increase2/1, GreaterThan2/1
  Detect Increase2/1 -> Logical Operator8/1
  GreaterThan2/1 -> Logical Operator8/2
  Logical Operator8/1 -> Logical Operator/3
  [VINP_FlashCTDLockSW_flg] -> GreaterThan2/2
  VBCM_CTDLockSW_flg/1 -> [VBCM_CTDLockSW_flg]
  [VBCM_TailgateHDSW_flg] -> Detect Increase3/1, GreaterThan3/1
  Detect Increase3/1 -> Logical Operator9/1
  [VINP_FlashTailgateHDSW_flg] -> GreaterThan3/2
  GreaterThan3/1 -> Logical Operator9/2
  VBCM_TailgateHDSW_flg/1 -> [VBCM_TailgateHDSW_flg]
  GreaterThan1/1 -> Logical Operator7/2
  Logical Operator7/1 -> Logical Operator/2
  [VINP_FlashTailgateSW_flg] -> GreaterThan1/2
  [VBCM_TailgateSW_flg] -> GreaterThan1/1, Detect Increase1/1
  Detect Increase1/1 -> Logical Operator7/1
  Logical Operator9/1 -> Logical Operator/4
  VINP_FlashHoodSW_flg/1 -> [VINP_FlashHoodSW_flg]
  VINP_FlashTailgateSW_flg/1 -> [VINP_FlashTailgateSW_flg]
  VINP_FlashCTDLockSW_flg/1 -> [VINP_FlashCTDLockSW_flg]
  VINP_FlashTailgateHDSW_flg/1 -> [VINP_FlashTailgateHDSW_flg]
  [task_time_s] -> Chart/2(task_time_s)
  Constant2/1 -> Chart/3(KBCM_SlpDebounceTime_s)
  [VBCM_SlpConditionMeet_flg] -> Chart/1(VBCM_SlpConditionMeet_flg)
  Logical Operator3/1 -> Goto11/1  "VBCM_WakeUp_flg"
  [VBCM_SleepReq_flg] -> VBCM_SleepReq_flg/1
  [VBCM_WakeUp_flg] -> VBCM_WakeUp_flg/1
  Logical Operator10/1 -> [VBCM_WakeUp_flg]
  Data Type Conversion/1 -> Logical Operator10/1, [VBCM_SleepReq_flg]  "VBCM_SleepReq_flg"
  Chart/1(VBCM_SleepReq_flg) -> Data Type Conversion/1
  Detect Increase/1 -> Logical Operator/6

== system bcm/BCM/BCM/CSW ==
  task_time_s : Inport
  VINP_CSWDimSwSta_flg : Inport  Port=2
  VINP_CSW2DimSwSta_flg : Inport  Port=3
  VINP_CSWPassSWSta_flg : Inport  Port=4
  VINP_CSW2PassSWSta_flg : Inport  Port=5
  VINP_CSWTurnSwSta_enum : Inport  Port=6
  VINP_CSW2TurnSwSta_enum : Inport  Port=7
  VINP_CSWFWipSwSta_enum : Inport  Port=8
  VINP_CSW2FWipSwSta_enum : Inport  Port=9
  VINP_CSWFWasSwSta_enum : Inport  Port=10
  VINP_CSW2FWasSwSta_enum : Inport  Port=11
  VINP_SASAngle_deg : Inport  Port=12
  VINP_TurnSwTimeSet_enum : Inport  Port=13
  VINP_LBeam_flg : Inport  Port=14
  VINP_CSW2RWIPWasSwSta_enum : Inport  Port=15
  VINP_CSWRWipIntSwSta_enum : Inport  Port=16
  VINP_CSWRWasSWSta_enum : Inport  Port=17
  Chart : Stateflow chart  TreatAsAtomicUnit=on
  Compare To Constant : simulink/Logic and Bit Operations/Compare To Constant  relop=<  const=3.0  OutDataTypeStr=boolean
  Compare To Constant1 : simulink/Logic and Bit Operations/Compare To Constant  relop=<  const=7  OutDataTypeStr=boolean
  Compare To Constant2 : simulink/Logic and Bit Operations/Compare To Constant  relop=<  const=3  OutDataTypeStr=boolean
  Compare To Constant3 : simulink/Logic and Bit Operations/Compare To Constant  relop=>=  const=5  OutDataTypeStr=boolean
  Compare To Constant4 : simulink/Logic and Bit Operations/Compare To Constant  relop=<  const=3.0  OutDataTypeStr=boolean
  Compare To Constant5 : simulink/Logic and Bit Operations/Compare To Constant  relop===  const=2  OutDataTypeStr=boolean
  Constant : Constant  Value=FALSE
  Constant1 : Constant  Value=45  OutDataTypeStr=int16
  Constant10 : Constant  Value=KBCM_TrunSWKeepTime5_s
  Constant11 : Constant  Value=2
  Constant12 : Constant  Value=KBCM_TrunSWKeepTime7_s
  Constant13 : Constant  Value=KBCM_TrunSWKeepTime3_s
  Constant2 : Constant  Value=TRUE
  Constant3 : Constant  Value=43  OutDataTypeStr=int16
  Constant4 : Constant  Value=FALSE
  Constant5 : Constant  Value=-45  OutDataTypeStr=int16
  Constant6 : Constant  Value=TRUE
  Constant7 : Constant  Value=-43  OutDataTypeStr=int16
  Constant8 : Constant  Value=FALSE
  Constant9 : Constant
  Data Type Conversion : DataTypeConversion  OutDataTypeStr=uint8
  Data Type Conversion1 : DataTypeConversion  OutDataTypeStr=uint16
  Data Type Conversion2 : DataTypeConversion  OutDataTypeStr=uint8
  Data Type Conversion3 : DataTypeConversion  OutDataTypeStr=uint8
  Detect Decrease : simulink/Logic and Bit Operations/Detect Decrease  vinit=0.0  OutDataTypeStr=boolean
  Detect Decrease1 : simulink/Logic and Bit Operations/Detect Decrease  vinit=0.0  OutDataTypeStr=boolean
  Detect Increase : simulink/Logic and Bit Operations/Detect Increase  vinit=0.0  OutDataTypeStr=boolean
  Detect Increase1 : simulink/Logic and Bit Operations/Detect Increase  vinit=0.0  OutDataTypeStr=boolean
  Divide : Product  Inputs=*/
  Logical Operator : Logic  Operator=NOT  AllPortsSameDT=off  OutDataTypeStr=boolean
  Logical Operator1 : Logic  AllPortsSameDT=off  OutDataTypeStr=boolean
  NOT : Logic  Operator=NOT  AllPortsSameDT=off  OutDataTypeStr=boolean
  OR : Logic  Operator=OR  AllPortsSameDT=off  OutDataTypeStr=boolean
  OR1 : Logic  Operator=OR  AllPortsSameDT=off  OutDataTypeStr=boolean
  Relational Operator : RelationalOperator  Operator=<  OutDataTypeStr=boolean  RndMeth=Simplest
  Relational Operator1 : RelationalOperator  Operator=>  OutDataTypeStr=boolean  RndMeth=Simplest
  Relational Operator2 : RelationalOperator  Operator=>  OutDataTypeStr=boolean  RndMeth=Simplest
  Relational Operator3 : RelationalOperator  Operator=<  OutDataTypeStr=boolean  RndMeth=Simplest
  Relational Operator4 : RelationalOperator  Operator===  OutDataTypeStr=boolean  RndMeth=Simplest
  Relational Operator5 : RelationalOperator  Operator===  OutDataTypeStr=boolean  RndMeth=Simplest
  Switch{,1..5} (6 alike) : Switch  Criteria=u2 > Threshold
  Switch{6..12} (7 alike) : Switch  Criteria=u2 ~= 0
  Unit Delay1 : UnitDelay  SampleTime=-1  HasFrameUpgradeWarning=on
  Unit Delay2 : UnitDelay  SampleTime=-1  HasFrameUpgradeWarning=on
  Unit Delay4 : UnitDelay  SampleTime=-1  HasFrameUpgradeWarning=on
  VBCM_DimSwSta_flg : Outport
  VBCM_PassSWSta_flg : Outport  Port=2
  VBCM_TurnSwSta_enum : Outport  Port=3
  VBCM_FWipSwSta_enum : Outport  Port=4
  VBCM_FWasSwSta_enum : Outport  Port=5
  VBCM_RWasSwSta_enum : Outport  Port=6
  VBCM_RWipIntSwSta_enum : Outport  Port=7
  wires:
  VINP_CSWDimSwSta_flg/1 -> OR/1
  Switch5/1 -> Switch4/3
  VINP_SASAngle_deg/1 -> Relational Operator1/2, Relational Operator2/2, Relational Operator3/2, Relational Operator/2
  Unit Delay2/1 -> Switch5/3
  Constant5/1 -> Relational Operator2/1
  Constant7/1 -> Relational Operator3/1
  Constant3/1 -> Relational Operator1/1
  Constant6/1 -> Switch4/1
  Relational Operator3/1 -> Switch5/2
  Detect Increase1/1 -> NOT/1
  Switch2/1 -> Unit Delay1/1, Detect Decrease/1
  Relational Operator1/1 -> Switch3/2
  Switch1/1 -> Switch/1
  VINP_CSW2TurnSwSta_enum/1 -> Compare To Constant3/1, Chart/1(VINP_CSW2TurnSwSta_enum)
  Switch6/1 -> [VBCM_WaitTimeSet_s]
  [LeftRelflg] -> Chart/2(LeftRelflg)
  Constant/1 -> Switch/3
  Constant1/1 -> Relational Operator/1
  Constant13/1 -> Switch7/3
  Switch7/1 -> Switch6/3
  Constant12/1 -> Switch7/1
  Constant10/1 -> Switch6/1
  [VINP_CSW2PassSWSta_flg] -> Detect Increase1/1
  Relational Operator2/1 -> Switch4/2
  OR/1 -> VBCM_DimSwSta_flg/1
  Constant8/1 -> Switch5/1
  Relational Operator/1 -> Switch2/2
  [RightRelflg] -> Chart/3(RightRelflg)
  Relational Operator5/1 -> Switch7/2
  Constant4/1 -> Switch3/1
  Detect Increase/1 -> Switch1/2
  Unit Delay1/1 -> Switch3/3
  Relational Operator4/1 -> Switch6/2
  Constant2/1 -> Switch2/1
  Switch4/1 -> Detect Decrease1/1, Unit Delay2/1
  VINP_CSW2FWipSwSta_enum/1 -> Compare To Constant1/1, Switch8/1
  VINP_CSW2DimSwSta_flg/1 -> Detect Increase/1
  VINP_TurnSwTimeSet_enum/1 -> [VINP_TurnSwTimeSet_enum]
  Switch8/1 -> VBCM_FWipSwSta_enum/1
  OR1/1 -> VBCM_PassSWSta_flg/1
  Switch3/1 -> Switch2/3
  VINP_CSW2PassSWSta_flg/1 -> [VINP_CSW2PassSWSta_flg], OR1/2
  [VINP_TurnSwTimeSet_enum] -> Relational Operator4/1
  [VINP_TurnSwTimeSet_enum] -> Relational Operator5/1
  VINP_LBeam_flg/1 -> Logical Operator1/1
  Switch/1 -> OR/2, Unit Delay4/1
  VINP_CSWPassSWSta_flg/1 -> OR1/1
  Compare To Constant1/1 -> Switch8/2
  VINP_CSWFWipSwSta_enum/1 -> Switch8/3
  VINP_CSWFWasSwSta_enum/1 -> Switch9/3
  Compare To Constant2/1 -> Switch9/2
  VINP_CSW2FWasSwSta_enum/1 -> Switch9/1, Compare To Constant2/1
  Switch9/1 -> VBCM_FWasSwSta_enum/1
  VINP_CSWTurnSwSta_enum/1 -> Switch10/1
  Compare To Constant3/1 -> Switch10/2
  Switch10/1 -> VBCM_TurnSwSta_enum/1
  Detect Decrease1/1 -> [LeftRelflg]
  Detect Decrease/1 -> [RightRelflg]
  Logical Operator1/1 -> Switch/2
  Unit Delay4/1 -> Logical Operator/1, Switch1/3
  Logical Operator/1 -> Switch1/1
  NOT/1 -> Logical Operator1/2
  Chart/1(CSW2TSw) -> Switch10/3
  VINP_CSW2RWIPWasSwSta_enum/1 -> Compare To Constant4/1, Compare To Constant5/1, Switch11/1, Compare To Constant/1
  Compare To Constant/1 -> Switch11/2
  VINP_CSWRWipIntSwSta_enum/1 -> Switch11/3
  Switch11/1 -> VBCM_RWipIntSwSta_enum/1
  Switch12/1 -> VBCM_RWasSwSta_enum/1
  Compare To Constant4/1 -> Switch12/2
  VINP_CSWRWasSWSta_enum/1 -> Switch12/3
  Data Type Conversion/1 -> Switch12/1
  Compare To Constant5/1 -> Data Type Conversion/1
  task_time_s/1 -> Divide/2
  [VBCM_WaitTimeSet_s] -> Divide/1
  Divide/1 -> Data Type Conversion1/1
  Data Type Conversion1/1 -> Chart/4(tset)
  Data Type Conversion2/1 -> Relational Operator4/2
  Constant9/1 -> Data Type Conversion2/1
  Constant11/1 -> Data Type Conversion3/1
  Data Type Conversion3/1 -> Relational Operator5/2

== system bcm/BCM/BCM/CenterDoorLock ==
  VINP_SetUnlockSingle_flg : Inport
  VBCM_AntitheftSta_enum : Inport  Port=2
  VBCM_AllDoorSW_flg : Inport  Port=3  OutDataTypeStr=boolean
  VTQD_DiagHCrash_flg : Inport  Port=4
  VPMM_PwrSta_enum : Inport  Port=5
  VINP_CentralDoorLockSW_flg : Inport  Port=6
  VBCM_BCMDoorLockSta_flg : Inport  Port=7
  VBCM_ATActCtrl_enum : Inport  Port=8
  VINP_AirBagFailCmd_flg : Inport  Port=9
  VINP_VehSpeed_kph : Inport  Port=10
  VINP_funAuto_flg : Inport  Port=11
  VINP_CDLUnlockButt_flg : Inport  Port=12  OutDataTypeStr=boolean
  VINP_CDLLockButt_flg : Inport  Port=13  OutDataTypeStr=boolean
  VTQD_CrashDetd_flg : Inport  Port=14
  VINP_CANMsgValidIVI2_flg : Inport  Port=15
  EEP_FuelDoorPos : Inport  Port=16
  EEP_LockSetting : Inport  Port=17
  VINP_FlashfUnlockSingle_flg : Inport  Port=18
  Chart : Stateflow chart  TreatAsAtomicUnit=on
  Data Type Conversion : DataTypeConversion  OutDataTypeStr=boolean
  Data Type Conversion1 : DataTypeConversion  OutDataTypeStr=boolean
  Detect Increase : simulink/Logic and Bit Operations/Detect Increase  vinit=0.0  OutDataTypeStr=boolean
  Switch : Switch  Criteria=u2 > Threshold
  Unit Delay : UnitDelay  SampleTime=-1  HasFrameUpgradeWarning=on
  VBCM_LockSetting_flg : Outport
  VBCM_FrChargingDoorCtrl_enum : Outport  Port=2
  VBCM_RrChargingDoorCtrl_enum : Outport  Port=3
  VBCM_CrashDetd_flg : Outport  Port=4
  VBCM_CTDCtrl_enum : Outport  Port=5
  DoorLockIND : Outport  Port=6
  VBCM_fVIGHandle_flg : Outport  Port=7
  VBCM_CTDLockSW_flg : Outport  Port=8
  VBCM_FuelDoorPos_flg : Outport  Port=9
  VBCM_DiagHCrash_flg : Outport  Port=10
  VBCM_fUnlockSingle_flg : Outport  Port=11
  wires:
  VBCM_AntitheftSta_enum/1 -> Chart/2(AntitheftSta)
  VINP_CDLUnlockButt_flg/1 -> Chart/11(CDL_Unlock_Butt)
  Chart/6(fVIGHandle) -> VBCM_fVIGHandle_flg/1  "VBCM_fVIGHandle_flg"
  Chart/1(LockSetting) -> VBCM_LockSetting_flg/1  "VBCM_LockSetting_flg"
  VINP_funAuto_flg/1 -> Chart/10(funAuto)
  VINP_VehSpeed_kph/1 -> Chart/9(VehSpeed)
  VINP_AirBagFailCmd_flg/1 -> Chart/8(AirBagFailCmd)
  VBCM_ATActCtrl_enum/1 -> Chart/7(ATLockCtrl)
  Chart/5(DoorLockIND) -> DoorLockIND/1  "VBCM_DoorLockIND_flg"
  VBCM_AllDoorSW_flg/1 -> Chart/3(AllDoorSW)
  Chart/2(FrChargingDoorCtrl) -> VBCM_FrChargingDoorCtrl_enum/1  "VBCM_FrChargingDoorCtrl_enum"
  Chart/3(RrChargingDoorCtrl) -> VBCM_RrChargingDoorCtrl_enum/1  "VBCM_RrChargingDoorCtrl_enum"
  VBCM_BCMDoorLockSta_flg/1 -> Chart/6(BCM_DoorLock_Sta)
  VINP_SetUnlockSingle_flg/1 -> Switch/1  "VINP_SetUnlockSingle_flg"
  Chart/4(CTDCtrl) -> VBCM_CTDCtrl_enum/1  "VBCM_CTDCtrl_enum"
  VINP_CDLLockButt_flg/1 -> Chart/12(CDL_Lock_Butt)
  [CTDLockSW] -> VBCM_CTDLockSW_flg/1  "VBCM_CTDLockSW_flg"
  Unit Delay/1 -> Switch/3
  Switch/1 -> Chart/1(SetUnlockSingle), Unit Delay/1
  VINP_CANMsgValidIVI2_flg/1 -> Switch/2
  VPMM_PwrSta_enum/1 -> [VPMM_PwrSta_enum]  "VPMM_PwrSta_enum"
  [VPMM_PwrSta_enum] -> Chart/4(PwrSta)
  VTQD_CrashDetd_flg/1 -> [VBCM_CrashDetd_flg]
  VINP_CentralDoorLockSW_flg/1 -> [CTDLockSW]  "VINP_CentralDoorLockSwSG09_flg"
  [CTDLockSW] -> Chart/5(CentralDoorLockSW)
  Detect Increase/1 -> Chart/13(CrashDetd)
  [VBCM_CrashDetd_flg] -> Detect Increase/1
  Data Type Conversion/1 -> VBCM_DiagHCrash_flg/1  "VBCM_DiagHCrash_flg"
  Data Type Conversion1/1 -> VBCM_CrashDetd_flg/1  "VBCM_CrashDetd_flg"
  VTQD_DiagHCrash_flg/1 -> Data Type Conversion/1
  [VBCM_CrashDetd_flg] -> Data Type Conversion1/1
  EEP_FuelDoorPos/1 -> Chart/14(EEP_FuelDoorPos)
  Chart/7(FuelDoorPos) -> VBCM_FuelDoorPos_flg/1  "VBCM_FuelDoorPos_flg"
  EEP_LockSetting/1 -> Chart/15(EEP_LockSetting)
  Chart/8(fUnlockSingle) -> VBCM_fUnlockSingle_flg/1  "VBCM_fUnlockSingle_flg"
  VINP_FlashfUnlockSingle_flg/1 -> Chart/16(VINP_FlashfUnlockSingle_flg)

== system bcm/BCM/BCM/Dimmer ==
  VINP_MFRDNBrightReq_pct : Inport
  VINP_IVIStatus_flg : Inport  Port=2
  VINP_IVINightModeSta_flg : Inport  Port=3
  VBCM_PosLamp_flag : Inport  Port=4
  VINP_CANMsgValidIVI2_flg : Inport  Port=5
  EEP_MFRDNBrightReq : Inport  Port=6
  BCMInitial : Inport  Port=7
  Chart : Stateflow chart  TreatAsAtomicUnit=on
      settings: PortSchema="{\"entries\":[{\"content\":{\"sides\":[{\"content\":{\"connectorIds\":[\"In4\",\"In1\",\"In2\",\"In3\"]},\"type\":\"ConnectorPlacement.EquallySpacedRectSide\",\"uuid\":\"076f305a-8f7e-4e65-8c9e-aa6699a69b21\"},{\"content\":{\"connectorIds\":[\"Out1\",\"Out2\"],\"side\":\"RIGHT\"},\"type\":\"ConnectorPlacement.EquallySpacedRectSide\",\"uuid\":\"bf947e95-3d60-4849-99c4-9fb941c8d282\"},{\"content\":{\"side\":\"TOP\"},\"type\":\"ConnectorPlacement.EquallySpacedRectSide\",\"uuid\":\"13c4efb7-da15-49ea-8253-a9d27aa3456c\"}]},\"type\":\"ConnectorPlacement.EquallySpacedConnector\",\"uuid\":\"7282b60f-551e-46a0-a3a5-beda89adbd0d\"}],\"packageUris\":[\"http://schema.mathworks.com/mf0/Connector/R2020b\"],\"version\":\"1.0\"}"
  Data Type Conversion1 : DataTypeConversion
  Switch1 : Switch  Criteria=u2 > Threshold
  Switch2 : Switch  Criteria=u2 > Threshold
  Switch3 : Switch  Criteria=u2 > Threshold
  Unit Delay : UnitDelay  SampleTime=-1  HasFrameUpgradeWarning=on
  Unit Delay1 : UnitDelay  SampleTime=-1  HasFrameUpgradeWarning=on
  VBCM_Dimmer_pct : Outport
  VBCM_DimmerEN_flg : Outport  Port=2
  VBCM_MFRDNBrightReq_pct : Outport  Port=3
  wires:
  VBCM_PosLamp_flag/1 -> Chart/3(PLamp)
  Chart/1(Dimmer) -> VBCM_Dimmer_pct/1  "VBCM_Dimmer_pct"
  VINP_IVIStatus_flg/1 -> Chart/1(IVI_Status)
  Chart/2(DimmerEN) -> VBCM_DimmerEN_flg/1  "VBCM_DimmerEN_flg"
  VINP_IVINightModeSta_flg/1 -> Switch1/1  "VINP_IVINightModeSta_flg"
  VINP_CANMsgValidIVI2_flg/1 -> Switch2/2, Switch1/2  "VINP_CANMsgValidIVI2_flg"
  Switch1/1 -> Unit Delay1/1, Chart/2(IVI_Night_Mode_Sta)
  Unit Delay1/1 -> Switch1/3
  BCMInitial/1 -> Switch3/2
  EEP_MFRDNBrightReq/1 -> Switch3/3
  Switch3/1 -> Data Type Conversion1/1, Unit Delay/1
  Switch2/1 -> Switch3/1
  Unit Delay/1 -> Switch2/3
  VINP_MFRDNBrightReq_pct/1 -> Switch2/1
  Data Type Conversion1/1 -> VBCM_MFRDNBrightReq_pct/1, Chart/4(MFRD_N_Bright_Req)  "VBCM_MFRDNBrightReq_pct"

== system bcm/BCM/BCM/ExteriorLight ==
  task_time_s : Inport
  VPMM_PwrSta_enum : Inport  Port=2
  VINP_HeadLampSW_enum : Inport  Port=3
  VINP_RFogLampSW_flg : Inport  Port=4
  VINP_BrakeSWGPIO_flg : Inport  Port=5
  VINP_CSWDimSw_flg : Inport  Port=6
  VINP_CSWPassSWSta_flg : Inport  Port=7
  VTQD_ShiftGearPosn_enum : Inport  Port=8
  VBCM_OutMode_enum : Inport  Port=9
  VINP_FollowMeSW_flg : Inport  Port=10
  VBCM_ATCtrl_enum : Inport  Port=11
  VINP_RLSLampSta_flg : Inport  Port=12
  VINP_ActBrkLampSta_flg : Inport  Port=13
  VINP_SRRODAWarnR_flg : Inport  Port=14
  VINP_SRRODAWarnL_flg : Inport  Port=15
  VINP_SRRBSDWarnR_flg : Inport  Port=16
  VINP_SRRBSDWarnL_flg : Inport  Port=17
  VINP_ForceLowBeam_enum : Inport  Port=18
  VINP_CANMsgValidIVI2_flg : Inport  Port=19
  VTQD_ReBrakeLPReq_flg : Inport  Port=20
  VINP_METERKPHCalcu_kph : Inport  Port=21
  VINP_DiagDRLOFF_flg : Inport  Port=22
  VINP_DiagFMHT_s : Inport  Port=23
  Chart : Stateflow chart  TreatAsAtomicUnit=on
      settings: PortSchema="{\"entries\":[{\"content\":{\"sides\":[{\"content\":{\"connectorIds\":[\"In1\",\"In2\",\"In3\",\"In4\",\"In5\",\"In6\",\"In7\",\"In8\",\"In9\",\"In10\",\"In11\",\"In12\",\"In13\",\"In14\",\"In15\",\"In16\",\"In17\",\"In18\",\"In21\",\"In19\",\"In22\",\"In20\"]},\"type\":\"ConnectorPlacement.EquallySpacedRectSide\",\"uuid\":\"34a74b70-26ca-4365-9514-cef344c89284\"},{\"content\":{\"connectorIds\":[\"Out1\",\"Out2\",\"Out3\",\"Out4\",\"Out5\",\"Out6\",\"Out7\",\"Out8\",\"Out9\",\"Out10\",\"Out11\",\"Out12\"],\"side\":\"RIGHT\"},\"type\":\"ConnectorPlacement.EquallySpacedRectSide\",\"uuid\":\"35b33564-17af-4a68-ba31-40ca81daf0a6\"},{\"content\":{\"connectorIds\":[],\"side\":\"TOP\"},\"type\":\"ConnectorPlacement.EquallySpacedRectSide\",\"uuid\":\"ba3f7f15-bc53-4e23-8d24-280f07cf706f\"}]},\"type\":\"ConnectorPlacement.EquallySpacedConnector\",\"uuid\":\"116adca9-6a34-4fe6-9115-066bd056288e\"}],\"packageUris\":[\"http://schema.mathworks.com/mf0/Connector/R2020b\"],\"version\":\"1.0\"}"
  Constant3 : Constant  Value=KBCM_ONDelayT_ms
  Divide : Product  Inputs=*/
  HeadLampErrorHanding : Subsystem
  Switch1 : Switch  Criteria=u2 > Threshold
  Unit Delay1 : UnitDelay  SampleTime=-1  HasFrameUpgradeWarning=on
  VBCM_PosLamp_flg : Outport
  VBCM_LBeam_flg : Outport  Port=2
  VBCM_HBeam_flg : Outport  Port=3
  VBCM_RrFogLamp_flg : Outport  Port=4
  VBCM_BrakeLamp_flg : Outport  Port=5
  VBCM_ReverseLamp_flg : Outport  Port=6
  VBCM_LDRL_flg : Outport  Port=7
  VBCM_RDRL_flg : Outport  Port=8
  VBCM_LBSD_flg : Outport  Port=9
  VBCM_RBSD_flg : Outport  Port=10
  VBCM_FollowMe_flg : Outport  Port=11
  VBCM_showup_flg : Outport  Port=12
  wires:
  Chart/11(VBCM_showup_flg) -> VBCM_showup_flg/1  "VBCM_showup_flg"
  VTQD_ReBrakeLPReq_flg/1 -> Chart/18(VTQD_ReBrakeLPReq_flg)
  VINP_DiagDRLOFF_flg/1 -> Chart/19(VBCM_DiagDRLOFF_flg)
  Unit Delay1/1 -> Switch1/3
  VINP_CANMsgValidIVI2_flg/1 -> Switch1/2, HeadLampErrorHanding/2(VINP_CANMsgValidIVI2_flg)  "VINP_CANMsgValidIVI2_flg"
  Switch1/1 -> Chart/3(VINP_RFogLampSW_flg), Unit Delay1/1
  Chart/6(VBCM_ReverseLamp_flg) -> VBCM_ReverseLamp_flg/1  "VBCM_ReverseLamp_flg"
  VTQD_ShiftGearPosn_enum/1 -> Chart/7(VTQD_ShiftGearPosn_enum)
  VINP_CSWDimSw_flg/1 -> Chart/5(VINP_CSWDimSw_flg)
  VBCM_ATCtrl_enum/1 -> Chart/10(VBCM_ATCtrl_enum)
  Chart/9(VBCM_LBSD_flg) -> VBCM_LBSD_flg/1  "VBCM_LBSD_flg"
  VINP_RLSLampSta_flg/1 -> Chart/11(VINP_RLSLampSta_flg)
  VINP_SRRBSDWarnR_flg/1 -> Chart/15(VINP_SRRBSDWarnR_flg)
  VINP_SRRBSDWarnL_flg/1 -> Chart/16(VINP_SRRBSDWarnL_flg)
  VINP_ActBrkLampSta_flg/1 -> Chart/12(VINP_ActBrkLampSta_flg)
  VINP_SRRODAWarnL_flg/1 -> Chart/14(VINP_SRRODAWarnL_flg)
  VINP_FollowMeSW_flg/1 -> Chart/9(VINP_FollowMeSW_flg)
  VINP_ForceLowBeam_enum/1 -> Chart/17(VINP_ForceLowBeam_enum)
  VINP_SRRODAWarnR_flg/1 -> Chart/13(VINP_SRRODAWarnR_flg)
  Chart/10(VBCM_RBSD_flg) -> VBCM_RBSD_flg/1  "VBCM_RBSD_flg"
  VBCM_OutMode_enum/1 -> Chart/8(VBCM_OutMode_enum)
  VINP_BrakeSWGPIO_flg/1 -> Chart/4(VINP_BrakeSWGPIO_flg)
  VINP_CSWPassSWSta_flg/1 -> Chart/6(VINP_CSWPassSWSta_flg)
  Chart/3(VBCM_HBeam_flg) -> VBCM_HBeam_flg/1  "VBCM_HBeam_flg"
  Chart/4(VBCM_RrFogLamp_flg) -> VBCM_RrFogLamp_flg/1  "VBCM_RrFogLamp_flg"
  VINP_RFogLampSW_flg/1 -> Switch1/1
  Chart/5(VBCM_BrakeLamp_flg) -> VBCM_BrakeLamp_flg/1  "VBCM_BrakeLamp_flg"
  Chart/2(VBCM_LBeam_flg) -> VBCM_LBeam_flg/1  "VBCM_LBeam_flg"
  Chart/7(VBCM_LDRL_flg) -> VBCM_LDRL_flg/1  "VBCM_LDRL_flg"
  Chart/8(VBCM_RDRL_flg) -> VBCM_RDRL_flg/1  "VBCM_RDRL_flg"
  VPMM_PwrSta_enum/1 -> Chart/1(VPMM_PwrSta_enum)
  Chart/1(VBCM_PosLamp_flg) -> VBCM_PosLamp_flg/1  "VBCM_PosLamp_flg"
  VINP_METERKPHCalcu_kph/1 -> Chart/21(VINP_METERKPHCalcu_kph)
  Constant3/1 -> Chart/22(KBCM_ONDelayT_ms)
  VINP_HeadLampSW_enum/1 -> HeadLampErrorHanding/1(VINP_HeadLampSW_enum)
  HeadLampErrorHanding/1(VBCM_HeadLampSW_enum) -> Chart/2(VINP_HeadLampSW_enum)
  Chart/12(VBCM_FollowMe_flg) -> VBCM_FollowMe_flg/1  "VBCM_FollowMe_flg"
  [task_time_s] -> Divide/2
  Divide/1 -> Chart/20(VBCM_DiagFMHT_s)
  task_time_s/1 -> [task_time_s]
  VINP_DiagFMHT_s/1 -> Divide/1
